simulink model "doc_design_iteration_viterbi_soft"  (R2014a)
settings: Solver=FixedStepDiscrete  StartTime=0.0  StopTime=inf  RelTol=1e-3
PreLoadFcn:
  | EbNo=0;
  | maxNumErrs=200;
  | maxNumBits=1e8;
libraries: commcnvcod2 x2, commdigbbndpm3 x2, commchan3 x1, commrandsrc2 x1, dspstat3 x1, dspmathops x1, commsink2 x1, dspquant2 x1
Description:
  | Parallel Concatenated Convolutional Coding: Turbo Codes
  | 
  | This demo model shows the layout of the Turbo Encoder as specified by 3GPP TS 36.212 v9.0
  | and the corresponding iterative Turbo Decoder.
  | 
  | The model can be configured to run with any one of the 188 block sizes supported by the standard
  | and is set to evaluate the BER performance of the code over an AWGN channel.
settings Model: FPTRunName=Active  Creator=The MathWorks Inc.
settings DataIOCC: SaveOutput=off  DSMLogging=off  SaveTime=off
settings OptimizationCC: ExpressionDepthLimit=2147483647  RollThreshold=2  SimCompilerOptimization=On
settings DebuggingCC: UnderspecifiedInitializationDetection=Classic  StateNameClashWarn=warning
settings GRTTargetCC: CombineOutputUpdateFcns=off  GRTInterface=on

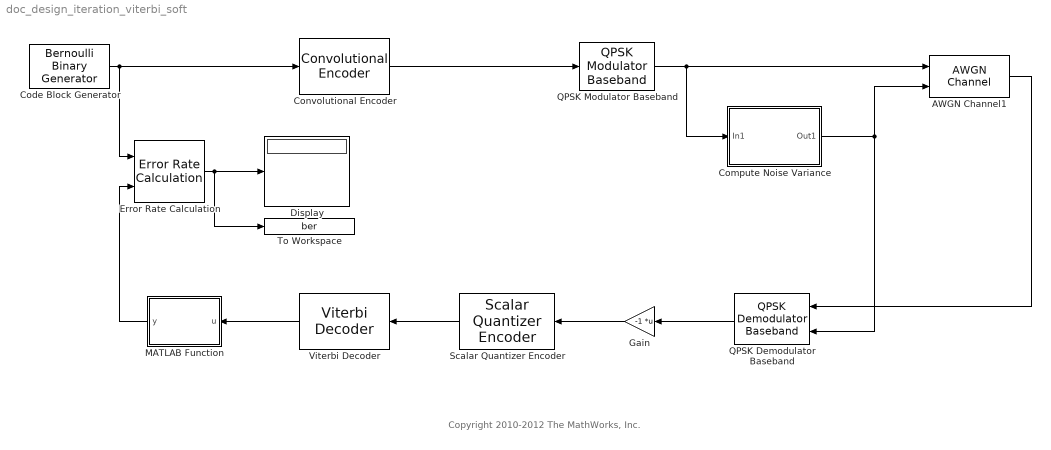
== system doc_design_iteration_viterbi_soft ==
  note: Copyright 2010-2012 The MathWorks, Inc.
  AWGN Channel1 : commchan3/AWGN Channel  InputProcessing=Columns as channels (frame based)  seed=67  noiseMode=Variance from port  EbNodB=10  EsNodB=15  SNRdB=10  bitsPerSym=1  Ps=1  Tsym=1e-6  variance=1
  Code Block Generator : commrandsrc2/Bernoulli Binary Generator  P=0.5  seed=12345  Ts=1/2040  frameBased=on  sampPerFrame=2040  orient=off  outDataType=boolean
  Compute Noise Variance : Subsystem
  Convolutional Encoder : commcnvcod2/Convolutional Encoder  trellis=poly2trellis(7, [171 133])  opMode=Terminate trellis by appending bits  DelayedResetAction=off  hasIniStPort=off  hasFinStPort=off  usePuncVector=off  punctureVector=[1; 1; 0; 1; 0; 1]  reset=Unused parameter value
  Display : Display
  Error Rate Calculation : commsink2/Error Rate Calculation  N=0  st_delay=0  cp_mode=Entire frame  subframe=[]  PMode=Port  WsName=ErrorVec1  RsMode2=off  stop=on  numErr=maxNumErrs  maxBits=maxNumBits
  Gain : Gain  Gain=-1  Multiplication=Matrix(K*u)
  MATLAB Function : MATLAB Function  TreatAsAtomicUnit=on
  QPSK Demodulator Baseband : commdigbbndpm3/QPSK Demodulator Baseband  Ph=pi/4  Dec=Gray  OutType=Bit  DecType=Log-likelihood ratio  VarSource=Port  Variance=1  outDtype1=boolean  outDtype2=Inherit via internal rule  derotateFactorWordLen=16
  QPSK Modulator Baseband : commdigbbndpm3/QPSK Modulator Baseband  InType=Bit  Enc=Gray  Ph=pi/4  outDtype=double  outWordLen=16  outUDDataType=sfix(16)  outFracLenMode=Best precision  outFracLen=15
  Scalar Quantizer Encoder : dspquant2/Scalar Quantizer Encoder  paramSrc=Specify via dialog  partType=Unbounded  BBoundary=[1:10]  UBoundary=[-7:7]  SearchMethod=Linear  tieBreakRule=Choose the lower index  outQU=off  outQError=off  codebook=[1.5:9.5]  outStatus=off  invalidin=Clip  idtype=uint8  roundingMode=Floor  overflowMode=off
  To Workspace : ToWorkspace  VariableName=ber  SampleTime=-1
      settings: MaxDataPoints=1
  Viterbi Decoder : commcnvcod2/Viterbi Decoder  trellis=poly2trellis(7, [171 133])  isPunctured=off  punctureVector=[1; 1; 0; 1; 0; 1]  erasures=off  dectype=Soft decision  runSigValErrCheck=off  nsdecb=4  smWordLength=16  tbdepth=34  opmode=Terminated  reset=off  outDataType=boolean  delayedResetAction=off
  wires:
  Code Block Generator/1 -> Error Rate Calculation/1, Convolutional Encoder/1
  Error Rate Calculation/1 -> Display/1, To Workspace/1
  Convolutional Encoder/1 -> QPSK Modulator Baseband/1
  Viterbi Decoder/1 -> MATLAB Function/1(u)
  MATLAB Function/1(y) -> Error Rate Calculation/2
  Scalar Quantizer Encoder/1 -> Viterbi Decoder/1
  QPSK Demodulator Baseband/1 -> Gain/1
  Gain/1 -> Scalar Quantizer Encoder/1
  AWGN Channel1/1 -> QPSK Demodulator Baseband/1
  QPSK Modulator Baseband/1 -> Compute Noise Variance/1(In1), AWGN Channel1/1
  Compute Noise Variance/1(Out1) -> QPSK Demodulator Baseband/2, AWGN Channel1/2

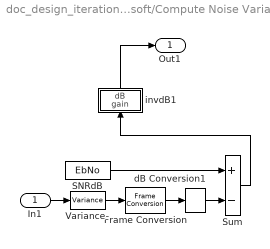
== system doc_design_iteration_viterbi_soft/Compute Noise Variance ==
  In1 : Inport
  Frame Conversion : FrameConversion  OutFrame=Sample-based
  SNRdB : Constant  Value=EbNo
  Sum : Sum  Inputs=+-  SaturateOnIntegerOverflow=on
  Variance : dspstat3/Variance  run=off  reset_popup=None  InputProcessing=Columns as channels (frame based)  directionMode=Each column  dimension=1  treatSBRowAsCol=on  roiEnable=off  roiType=Rectangles  roiPortion=Entire ROI  roiOutput=Individual statistics for each ROI  roiFlag=off  roundingMode=Floor  overflowMode=off
  dB Conversion1 : dspmathops/dB Conversion  dBtype=dB  intype=Power  R=1  fuzz=on
  invdB1 : Subsystem
      mask Display: disp('1/invdB')
  Out1 : Outport
  wires:
  In1/1 -> Variance/1
  invdB1/1(dB) -> Out1/1
  dB Conversion1/1 -> Sum/2
  Variance/1 -> Frame Conversion/1
  Sum/1 -> invdB1/1(gain)
  SNRdB/1 -> Sum/1
  Frame Conversion/1 -> dB Conversion1/1

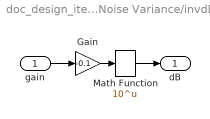
== system doc_design_iteration_viterbi_soft/Compute Noise Variance/invdB1 ==
  gain : Inport
  Gain : Gain  Gain=-0.1  SaturateOnIntegerOverflow=on  OutDataTypeStr=Inherit: Same as input  ParamDataTypeStr=Inherit: Same as input
  Math Function : Math  Operator=10^u  SaturateOnIntegerOverflow=on
  dB : Outport
  wires:
  Gain/1 -> Math Function/1
  gain/1 -> Gain/1
  Math Function/1 -> dB/1

== matlab function doc_design_iteration_viterbi_soft/MATLAB Function ==
  data: u input; y output boolean
function y = fcn(u)
%#codegen

y = u(1:2040);
